simulink model "power_battery_Lead_Acid_2015"  (R2015b)
settings: Solver=ode23s  StartTime=0.0  StopTime=40301  RelTol=1e-4
undefined symbols (not defined in the file or in its folder): Batt, BatteryCback, BatteryLoadFcn, gcbh, sps_rtmsupport
libraries: powerlib x5, spsBatteryModel x1
Description:
  | Copyright 2008-2011 The MathWorks, Inc.
settings Model: Creator=MathWorks  LastModifiedBy=gmiglio
settings DataIOCC: LimitDataPoints=off  SaveFormat=Array  SignalLoggingSaveFormat=ModelDataLogs
settings OptimizationCC: ExpressionDepthLimit=2147483647  InitFltsAndDblsToZero=on
settings DebuggingCC: UnderspecifiedInitializationDetection=Classic  MergeDetectMultiDrivingBlocksExec=none  SignalResolutionControl=TryResolveAllWithWarning  FcnCallInpInsideContextMsg=UseLocalSettings  StateNameClashWarn=warning
settings HardwareCC: ProdBitPerPointer=32  ProdLargestAtomicFloat=None  ProdIntDivRoundTo=Undefined  ProdEndianess=Unspecified  ProdWordSize=32  ProdHWDeviceType=32-bit Generic
settings GRTTargetCC: GeneratePreprocessorConditionals=Disable all  CombineOutputUpdateFcns=off  GRTInterface=on
settings ConfigComp: CovModelRefEnable=Off

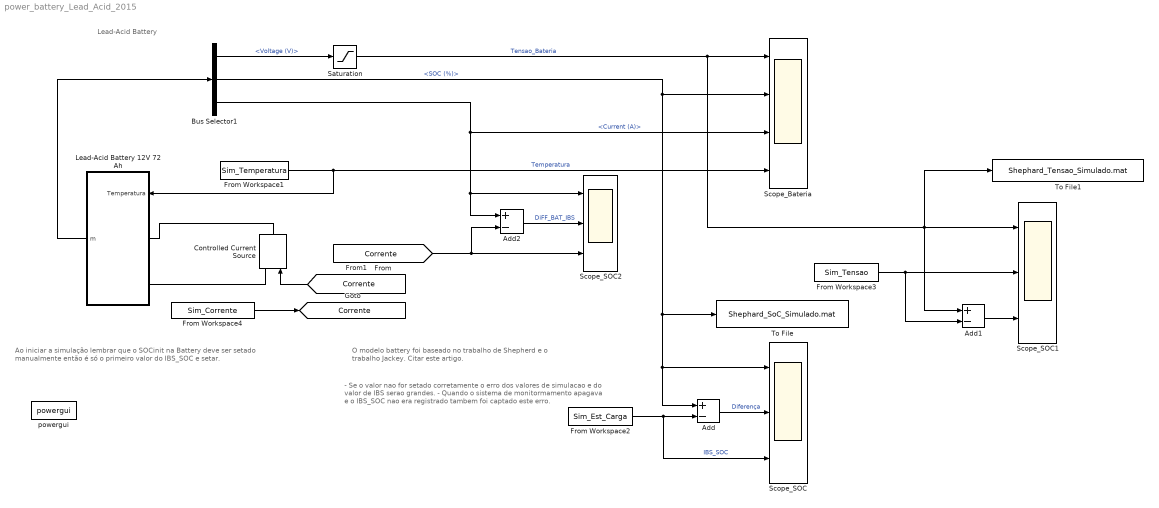
== system power_battery_Lead_Acid_2015 ==
  note: O modelo battery foi baseado no trabalho de Shepherd e o
      | trabalho Jackey. Citar este artigo.
  note: Ao iniciar a simulação lembrar que o SOCinit na Battery deve ser setado
      | manualmente então é só o primeiro valor do IBS_SOC e setar.
  note: Lead-Acid Battery
  note: - Se o valor nao for setado corretamente o erro dos valores de simulacao
      | e do valor de IBS serao grandes.
      | - Quando o sistema de monitormamento apagava e o IBS_SOC nao era
      | registrado tambem foi captado este erro.
  Add : Sum  Inputs=+-
  Add1 : Sum  Inputs=+-
  Add2 : Sum  Inputs=+-
  Bus Selector1 : BusSelector  OutputSignals=Voltage (V),SOC (%),Current (A)
  Controlled Current Source : powerlib/Electrical Sources/Controlled Current Source  Initialize=off  Source_Type=AC  Amplitude=0  Phase=0  Frequency=0  Measurements=Current
  From Workspace1 : FromWorkspace  VariableName=Sim_Temperatura  SampleTime=0
  From Workspace2 : FromWorkspace  VariableName=Sim_Est_Carga  SampleTime=0
  From Workspace3 : FromWorkspace  VariableName=Sim_Tensao  SampleTime=0
  From Workspace4 : FromWorkspace  VariableName=Sim_Corrente  SampleTime=0  Interpolate=off  OutputAfterFinalValue=Setting to zero
  Lead-Acid Battery 12V 72 Ah : Subsystem  AncestorBlock=electricdrivelib/Extra Sources/Battery  DialogController=POWERSYS.PowerSysDialog  LoadFcn=sps_rtmsupport('LoadFcn',gcbh); BatteryLoadFcn(gcb)  InitFcn=BatteryCback(gcb,1)  StartFcn=sps_rtmsupport('StartFcn',gcbh);  StopFcn=sps_rtmsupport('StopFcn',gcbh);  mask(Battery){BatType=Lead-Acid, ShowTempParam=off, ThermalPreset=no, NomV=12, NomQ=60, SOC=81, Batt_Tr=0.5, PresetModel=on, MaxQ=62.5, FullV=13.0658, Dis_rate=12, R=0.002, Normal_OP=18.6167, expZone=[12.2171          0.2], current=[3.6 7.2 14.4], Units=Ampere-hour, Tci=20, NomT=20, T2=-30, MaxQ2=4.8, FullV2=7.1, Normal_OP2=5.72, expZone2=[6.58  1], Rca=0.6, ti=1000}
      mask prompts: BatType "Type:"; ShowTempParam "Simulate temperature effects"; ThermalPreset "Use a preset battery:"; NomV "Nominal voltage (V)"; NomQ "Rated capacity (Ah)"; SOC "Initial state-of-charge (%)"; Batt_Tr "Battery response time (s)"; PresetModel "Determined from the nominal parameters of the battery"; MaxQ "Maximum capacity (Ah)"; FullV "Fully charged voltage (V)"; Dis_rate "Nominal discharge current (A)"; R "Internal resistance (Ohms)"; Normal_OP "Capacity (Ah) at nominal voltage"; expZone "Exponential zone [Voltage (V), Capacity (Ah)]"; current "Discharge current [i1, i2, i3,...] (A)"; Tci "Initial cell temperature (deg. C)"; NomT "Nominal ambient temperature T1 (deg. C)"; T2 "Second ambient temperature T2 (deg. C)"; MaxQ2 "Maximum capacity (Ah)"; FullV2 "Initial discharge voltage (V)"; Normal_OP2 "Voltage at 90% maximum capacity (V)"; expZone2 "Exponential zone [Voltage (V), Capacity (Ah)]"; Rca "Thermal resistance, cell-to-ambient (deg. C/W)"; ti "Thermal time constant, cell-to-ambient (s)"
      mask help: Implements a generic battery that model most popular battery types. Temperature effects can be specified for Lithium-Ion battery type.
      mask init:
      | block = gcb;
      | BatteryCback(block,3)
      | [Batt BT, WantBlockChoice, Ts] = BatteryParam(NomV,NomQ,MaxQ,FullV,Dis_rate,R,Normal_OP,expZone,block,0);
      | powericon('SetInternalModels','set',block,WantBlockChoice);
      | BatteryCback(block,1); %sps_rtmsupport('parametereditingmodes',gcbh, [1,2,3,8,16]);
      | if Batt.sel_T
      |     set_param([block,'/','Output'],'OverrideUsingVariant','OutputwithT');
      | else
      |     set_param([block,'/','Output'],'OverrideUsingVariant','OutputwithoutT');
      | end
      settings: CopyFcn=sps_rtmsupport('CopyFcn',gcbh);  DeleteFcn=sps_rtmsupport('DeleteFcn',gcbh);  UndoDeleteFcn=sps_rtmsupport('UndoDeleteFcn',gcbh);  ModelCloseFcn=sps_rtmsupport('ModelCloseFcn',gcbh);  PreSaveFcn=sps_rtmsupport('PreSaveFcn',gcbh);  PostSaveFcn=sps_rtmsupport('PostSaveFcn',gcbh);  NameChangeFcn=sps_rtmsupport('NameChangeFcn',gcbh);  PreCopyFcn=sps_rtmsupport('PreCopyFcn',gcbh);  OpenFcn=sps_rtmsupport('OpenFcn',gcbh, [1,2,3,8,16]); open_system(gcb,'Mask')  CloseFcn=sps_rtmsupport('CloseFcn',gcbh);  PreDeleteFcn=sps_rtmsupport('PreDeleteFcn',gcbh);
      mask Help: helpview(psbhelp)
      mask TypeOptions BatType: Lead-Acid | Lithium-Ion | Nickel-Cadmium | Nickel-Metal-Hydride
      mask Callback BatType: BatteryCback(gcb,1)
      mask Callback ShowTempParam: BatteryCback(gcb,1)
      mask TypeOptions ThermalPreset: no | 3.3V  2.3Ah  (LiFePO4) | 3.6V  2050mAh   (LiCoO2) | 3.6V  2.0Ah | 3.6V  3.6Ah  (LiNiO2) | 3.6V  4.5Ah | 3.6V  48Ah  (LiNiO2) | 3.7V  4.4Ah | 7.4V  5.4Ah  (LiCoO2) | 11.1V  6600mAh  (LiCoO2) | 12.8V  40Ah  (LiFeMgPO4)
      mask Callback ThermalPreset: BatteryCback(gcb,1)
      mask Callback PresetModel: BatteryCback(gcb,1)
      mask TypeOptions Units: Ampere-hour | Time
      mask Callback ti: sps_rtmsupport('parametereditingmodes',gcbh, [1,2,3,8,16]);
      mask DialogControl Tempcontainer Prompt: Temperature
      mask DialogControl Container9 Prompt: Display characteristics
      mask DialogControl PlotButton Prompt: Plot
      mask DialogControl PlotButton Callback: BatteryCback(gcb,0)
      mask DialogControl Container7 Prompt: Discharge parameters at T2
      mask DialogControl Container8 Prompt: Thermal response
      mask Display:
      | patch([BT.X1 BT.X1m],[BT.Y1 BT.Y1m],BT.color1);
      | patch(BT.X3,BT.Y3,BT.color2);
      | plot([BT.X1 BT.X1m BT.X2 BT.X2m BT.X3 BT.X4],[BT.Y1 BT.Y1m BT.Y2 BT.Y2m BT.Y3 BT.Y4]);
      | plot(-100,-60,60,50,[BT.X(1) BT.X(1)],[BT.bas BT.haut],[BT.X(2) BT.X(2)],[BT.haut BT.bas],BT.dim_Xsin,4*sin(BT.dim_sin)+BT.haut,BT.dim_Xsin,-4*sin(BT.dim_sin)+BT.haut,BT.dim_Xsin,-4*sin(BT.dim_sin)+BT.bas,BT.dim_Xtop,sin(BT.dim_top)+BT.haut+4,BT.dim_Xtop,-sin(BT.dim_top)+BT.haut+4,BT.dim_Xtop,-sin(BT.dim_top)+BT.haut,[BT.TopX(2),BT.TopX(2)],[BT.haut,BT.haut+4],[BT.TopX(1),BT.TopX(1)],[BT.haut+4,BT.haut]);plot(BT.dim_Xsin,-5*sin(BT.dim_sin)+20);
      | port_label('lconn',1,'+');
      | port_label('lconn',2,'_');
      | color('blue');
      | port_label('output',1,'m');
      | 
      | if Batt.sel_T
      |     port_label('input',1,'Ta');
      | end
  Saturation : Saturate  UpperLimit=16.5  LowerLimit=0
  Scope_Bateria : Scope  NumInputPorts=4
  Scope_SOC : Scope  NumInputPorts=3
  Scope_SOC1 : Scope  NumInputPorts=3
  Scope_SOC2 : Scope  NumInputPorts=3
  To File : ToFile  Filename=Shephard_SoC_Simulado.mat  MatrixName=Shephard_SoC_Simulado  SaveFormat=Timeseries
  To File1 : ToFile  Filename=Shephard_Tensao_Simulado.mat  MatrixName=Shephard_Tensao_Simulado  SaveFormat=Timeseries
  powergui : powerlib/powergui  SimulationMode=Continuous  SolverType=Tustin  SampleTime=0.001  frequency=60  SPID=off  DisableSnubberDevices=off  DisableRonSwitches=off  DisableVfSwitches=off  SwTol=0  DisplayEquations=off  Interpol=off  ExternalGateDelay=off  methode=off  Ts=0  FunctionMessages=off  echomessages=off  HookPort=off  EnableUseOfTLC=off  x0status=blocks  frequencyindice=0  Pbase=100e6  ErrMax=1e-4  Iterations=50  UnitsV=kV  UnitsW=MW  buscounter=0  RestoreLinks=warning  ResistiveCurrentMeasurement=off  Frange=[0:2:500]  Ylog=off  Xlog=on  ShowGrid=off  save=off  variable=ZData  structure=0  ZoomFFT=on  StartTime=0.0  cycles=1  DisplayStyle=1  fundamental=60  FreqAxis=off  MaxFrequency=1000  frequencyindicesteady=1  RmsSteady=1  display=off
  tag scope: Corrente=global
  wires:
  Lead-Acid Battery 12V 72 Ah/1(m) -> Bus Selector1/1
  Bus Selector1/2 -> To File/1, Add/1, Scope_SOC/1, Scope_Bateria/2  "<SOC (%)>"
  Bus Selector1/1 -> Saturation/1  "<Voltage (V)>"
  Saturation/1 -> To File1/1, Add1/1, Scope_SOC1/1, Scope_Bateria/1  "Tensao_Bateria"
  [Corrente] -> Add2/2, Scope_SOC2/3
  From Workspace2/1 -> Scope_SOC/3, Add/2  "IBS_SOC"
  Add/1 -> Scope_SOC/2  "Diferença"
  From Workspace3/1 -> Scope_SOC1/2, Add1/2
  Add1/1 -> Scope_SOC1/3
  From Workspace1/1 -> Lead-Acid Battery 12V 72 Ah/1(Temperatura), Scope_Bateria/4  "Temperatura"
  Bus Selector1/3 -> Add2/1, Scope_SOC2/1, Scope_Bateria/3  "<Current (A)>"
  Add2/1 -> Scope_SOC2/2  "DiFF_BAT_IBS"
  From Workspace4/1 -> [Corrente]
  [Corrente] -> Controlled Current Source/1
  connections:
  Controlled Current Source/LConn1 -- Lead-Acid Battery 12V 72 Ah/LConn2
  Controlled Current Source/RConn1 -- Lead-Acid Battery 12V 72 Ah/LConn1

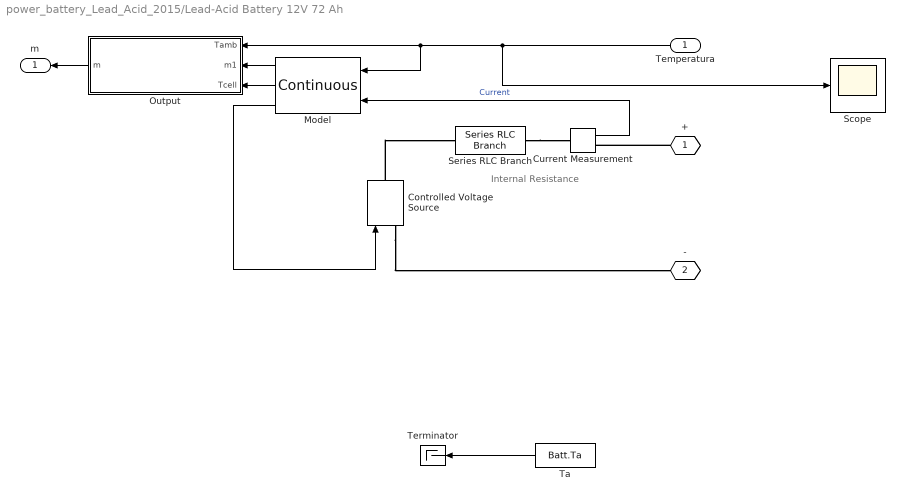
== system power_battery_Lead_Acid_2015/Lead-Acid Battery 12V 72 Ah ==
  note: Internal Resistance
  Temperatura : Inport
  Controlled Voltage Source : powerlib/Electrical Sources/Controlled Voltage Source  Initialize=on  Source_Type=AC  Amplitude=0  Phase=0  Frequency=0  Measurements=None
  Current Measurement : powerlib/Measurements/Current Measurement  PhasorSimulation=off  OutputType=Complex  PSBequivalent=0
  Model : spsBatteryModel/Continuous
  Output : Subsystem  Variant=on  OverrideUsingVariant=OutputwithoutT
  Scope : Scope
  Series RLC Branch : powerlib/Elements/Series RLC Branch  LConnTagsString=__new0  RConnTagsString=__new0  BranchType=R  Resistance=Batt.R  Inductance=1e-3  SetiL0=off  InitialCurrent=0  Capacitance=1e-6  Setx0=off  InitialVoltage=0  Measurements=None
  Ta : Constant  Value=Batt.Ta
  Terminator : Terminator
  + : PMIOPort  Tag=PMCPort  Port=1  Side=Left
  - : PMIOPort  Tag=PMCPort  Port=2  Side=Left
  m : Outport
  wires:
  Output/1(m) -> m/1
  Model/1 -> Output/2(m1)
  Current Measurement/1 -> Model/2  "Current"
  Temperatura/1 -> Scope/1, Output/1(Tamb), Model/1
  Model/2 -> Output/3(Tcell)
  Model/3 -> Controlled Voltage Source/1
  Ta/1 -> Terminator/1
  connections:
  +/RConn1 -- Current Measurement/RConn1
  Controlled Voltage Source/LConn1 -- -/RConn1
  Controlled Voltage Source/RConn1 -- Series RLC Branch/LConn1
  Series RLC Branch/RConn1 -- Current Measurement/LConn1

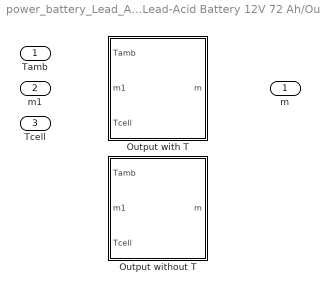
== system power_battery_Lead_Acid_2015/Lead-Acid Battery 12V 72 Ah/Output ==
  Tamb : Inport
  m1 : Inport  Port=2
  Tcell : Inport  Port=3
  Output with T : Subsystem  VariantControl=OutputwithT
  Output without T : Subsystem  VariantControl=OutputwithoutT
  m : Outport

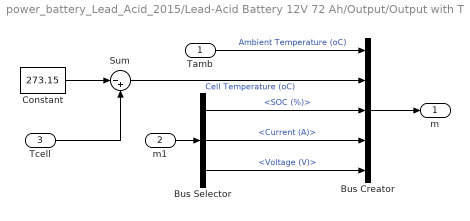
== system power_battery_Lead_Acid_2015/Lead-Acid Battery 12V 72 Ah/Output/Output with T ==
  Tamb : Inport
  m1 : Inport  Port=2
  Tcell : Inport  Port=3
  Bus Creator : BusCreator  Inputs=5
  Bus Selector : BusSelector  OutputSignals=SOC (%),Current (A),Voltage (V)
  Constant : Constant  Value=273.15
  Sum : Sum  Inputs=|-+
  m : Outport
  wires:
  Sum/1 -> Bus Creator/2  "Cell Temperature (oC)"
  Tcell/1 -> Sum/2
  Constant/1 -> Sum/1
  Tamb/1 -> Bus Creator/1  "Ambient Temperature (oC)"
  Bus Selector/3 -> Bus Creator/5  "<Voltage (V)>"
  Bus Selector/1 -> Bus Creator/3  "<SOC (%)>"
  Bus Selector/2 -> Bus Creator/4  "<Current (A)>"
  Bus Creator/1 -> m/1
  m1/1 -> Bus Selector/1

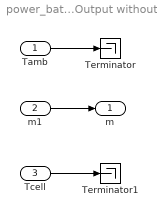
== system power_battery_Lead_Acid_2015/Lead-Acid Battery 12V 72 Ah/Output/Output without T ==
  Tamb : Inport
  m1 : Inport  Port=2
  Tcell : Inport  Port=3
  Terminator : Terminator
  Terminator1 : Terminator
  m : Outport
  wires:
  m1/1 -> m/1
  Tcell/1 -> Terminator1/1
  Tamb/1 -> Terminator/1
